simulink model "irp_model"  (R2016a)
settings: Solver=ode1  StartTime=0  StopTime=inf  FixedStep=0.001  RelTol=1e-3
PostLoadFcn:
  | , if any(exist('dsrtsu_mdlpostloadfcn', 'file') == [2, 3, 6]), try dsrtsu_mdlpostloadfcn('Execute', bdroot); catch fprintf('Error in PostLoadFcn (dsrtsu_mdlpostloadfcn) for model "%s":\n %s\n', bdroot, lasterr); end, end,
libraries: rtilibm x3, simulink_extras x3
settings Model: DSRTSU_INTERNAL_RTI_VER=460  DSRTSU_INTERNAL_RTI_TYPE=rti1005  DSRTSU_INTERNAL_RTIFPGA=50  Creator=k18w1400a  LastModifiedBy=Dominik
settings DataIOCC: LimitDataPoints=on  SaveFormat=Array
settings OptimizationCC: BlockReduction=off  BooleanDataType=off  OptimizeBlockIOStorage=off  BufferReuse=off  GlobalBufferReuse=off  ExpressionFolding=off  LocalBlockOutputs=off
settings HardwareCC: ProdBitPerPointer=32  ProdLargestAtomicFloat=None  ProdEndianess=BigEndian  ProdWordSize=32  ProdHWDeviceType=Generic->Custom  TargetIntDivRoundTo=Zero  TargetEndianess=BigEndian  TargetHWDeviceType=Generic->Custom
settings ModelReferenceCC: PropagateSignalLabelsOutOfModel=off
settings RTWCC: SystemTargetFile=rti1005.tlc  MakeCommand=make_rti  TemplateMakefile=rti1005.tmf  Description=dSPACE DS1005 Hardware Platform
settings STFCustomTargetCC: ParMdlRefBuildCompliant=on  GeneratePreprocessorConditionals=Disable all  SystemTargetFile=rti1005.tlc
settings GRTTargetCC: CompOptLevelCompliant=off  ConcurrentExecutionCompliant=off  CombineOutputUpdateFcns=off  MatFileLogging=off  CPPClassGenCompliant=off  GRTInterface=on  UseToolchainInfoCompliant=off  ExtModeMexFile=noextcomm
settings ConfigComp: CovModelRefEnable=Off

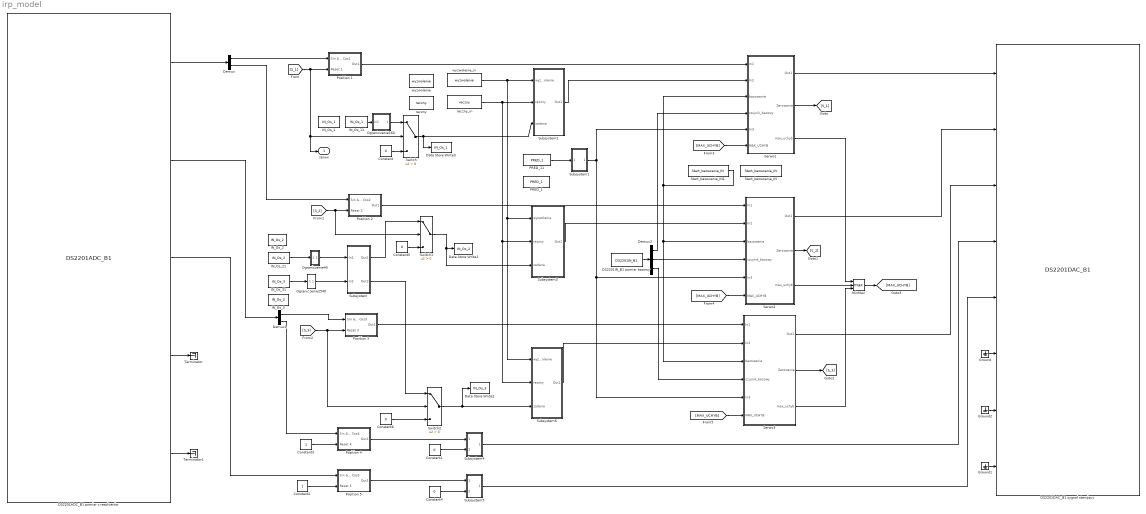
== system irp_model ==
  Constant{,1,4..6} (5 alike) : Constant  Value=0
  Constant2 : Constant
  Constant3 : Constant
  DS2201ADC_B1 pomiar z resolverów : rtilibm/DS2201/DS2201ADC_B1  BoardNo=1  channelNo1=[1 2 3 4]  channelNo2=[5 6 7 8]  channelNo3=[9 10]  channelNo4=-1  channelNo5=-1  DialogFcn=gui2201adc  UnitName={'DS2201ADC_B'}  UnitValues={ 1 }  DSProperties=struct('RTI',struct('Version',uint32(1),'BlockType',struct('isSLSource',uint8(1),'isSLSink',uint8(0),'isHWSource',uint8(1),'isHWSink',uint8(0),'isSetup',uint8(0),'isInline',uint8(1),'isNonInline',uint8(0),'isInterrupt',uint8(0),'isChannelwise',uint8(0)),'IOBoardType','DS2201','UnitType','ADC','Identifier','ADCMUX','DialogType','ML','BlockSet','NONE','SlaveProcessor','NONE'))
  DS2201DAC_B1 sygnał sterujący : rtilibm/DS2201/DS2201DAC_B1  BoardNo=1  IOErrorMode=[0 0]  InitValue=[0 0 0 0 0 0 0 0]  TermMode=[1 1 1 1 1 1 1 1]  TermValue=[0 0 0 0 0 0 0 0]  DialogFcn=gui2201dac  UnitName={'DS2201DAC_B'}  UnitValues={ 1 }  DSProperties=struct('RTI',struct('Version',uint32(1),'BlockType',struct('isSLSource',uint8(0),'isSLSink',uint8(1),'isHWSource',uint8(0),'isHWSink',uint8(1),'isSetup',uint8(0),'isInline',uint8(1),'isNonInline',uint8(0),'isInterrupt',uint8(0),'isChannelwise',uint8(0)),'IOBoardType','DS2201','UnitType','DAC','Identifier','DAC','DialogType','ML','BlockSet','NONE','SlaveProcessor','NONE'))
  DS2201IN_B1 pomiar bazowy : rtilibm/DS2201/DS2201IN_B1  BoardNo=1  ChannelNos=[1 2 3]  DialogFcn=gui2201in  UnitName={ 'DS2201IN_B' }  UnitValues={ 1 }  DSProperties=struct('RTI',struct('Version',uint32(1),'BlockType',struct('isSLSource',uint8(1),'isSLSink',uint8(0),'isHWSource',uint8(1),'isHWSink',uint8(0),'isSetup',uint8(0),'isInline',uint8(1),'isNonInline',uint8(0),'isInterrupt',uint8(0),'isChannelwise',uint8(0)),'IOBoardType','DS2201','UnitType','BIT','Identifier','BITIN','DialogType','ML','BlockSet','NONE','SlaveProcessor','NONE'))
  Data Store Write1 : DataStoreWrite  DataStoreName=IN_Os_2
  Data Store Write2 : DataStoreWrite  DataStoreName=IN_Os_3
  Data Store Write3 : DataStoreWrite  DataStoreName=IN_Os_1
  Demux : Demux  Outputs=2
  Demux1 : Demux  Outputs=2
  Demux2 : Demux  Outputs=3
  Ground : Ground
  Ground1 : Ground
  Ground2 : Ground
  "IN_Os_1 " : DataStoreMemory  DataStoreName=IN_Os_1  ReadBeforeWriteMsg=warning  WriteAfterWriteMsg=warning  WriteAfterReadMsg=warning  ShowAdditionalParam=off
  IN_Os_11 : DataStoreRead  DataStoreName=IN_Os_1
  "IN_Os_2 " : DataStoreMemory  DataStoreName=IN_Os_2  ReadBeforeWriteMsg=warning  WriteAfterWriteMsg=warning  WriteAfterReadMsg=warning  ShowAdditionalParam=off
  IN_Os_21 : DataStoreRead  DataStoreName=IN_Os_2
  "IN_Os_3 " : DataStoreMemory  DataStoreName=IN_Os_3  ReadBeforeWriteMsg=warning  WriteAfterWriteMsg=warning  WriteAfterReadMsg=warning  ShowAdditionalParam=off
  IN_Os_31 : DataStoreRead  DataStoreName=IN_Os_3
  MinMax : MinMax  Function=max  Inputs=3
  Ograniczenie160 : Subsystem
  Ograniczenie2540 : Subsystem
  Ograniczenie40 : Subsystem
  "PRED_1 " : DataStoreMemory  DataStoreName=PRED_1  ReadBeforeWriteMsg=warning  WriteAfterWriteMsg=warning  WriteAfterReadMsg=warning  InitialValue=50  ShowAdditionalParam=off
  "PRED_11 " : DataStoreRead  DataStoreName=PRED_1
  Position 1 : Subsystem
  Position 2 : Subsystem
  Position 3 : Subsystem
  Position 4 : Subsystem
  Position 5 : Subsystem
  Serwo1 : Subsystem
  Serwo2 : Subsystem
  Serwo3 : Subsystem
  "Start_bazowania_IN " : DataStoreMemory  DataStoreName=Start_bazowania_IN  ReadBeforeWriteMsg=warning  WriteAfterWriteMsg=warning  WriteAfterReadMsg=warning  ShowAdditionalParam=off
  Start_bazowania_IN1 : DataStoreRead  DataStoreName=Start_bazowania_IN
  Subsystem : Subsystem
  Subsystem1 : Subsystem
  Subsystem2 : Subsystem
  Subsystem3 : Subsystem
  Subsystem4 : Subsystem
  Subsystem5 : Subsystem
  Subsystem6 : Subsystem
  Switch : Switch  Criteria=u2 > Threshold
  Switch1 : Switch  Criteria=u2 > Threshold
  Switch2 : Switch  Criteria=u2 > Threshold
  Terminator : Terminator
  Terminator1 : Terminator
  "reczny " : DataStoreMemory  DataStoreName=reczny  ReadBeforeWriteMsg=warning  WriteAfterWriteMsg=warning  WriteAfterReadMsg=warning  ShowAdditionalParam=off
  "reczny_in " : DataStoreRead  DataStoreName=reczny
  "wyzwolenie " : DataStoreMemory  DataStoreName=wyzwolenie  ReadBeforeWriteMsg=warning  WriteAfterWriteMsg=warning  WriteAfterReadMsg=warning  ShowAdditionalParam=off
  "wyzwolenie_in " : DataStoreRead  DataStoreName=wyzwolenie
  zerow : Outport
  wires:
  Demux/1 -> Position 1/1(Sin && Cos1)
  Demux/2 -> Position 2/1(Sin && Cos2)
  DS2201ADC_B1 pomiar z resolverów/2 -> Demux1/1
  DS2201ADC_B1 pomiar z resolverów/1 -> Demux/1
  Demux1/1 -> Position 3/1(Sin && Cos3)
  Demux1/2 -> Position 4/1(Sin && Cos4)
  Constant3/1 -> Position 4/2(Reset 4)
  DS2201ADC_B1 pomiar z resolverów/3 -> Position 5/1(Sin && Cos5)
  Constant2/1 -> Position 5/2(Reset 5)
  IN_Os_21/1 -> Ograniczenie40/1(In1)
  IN_Os_31/1 -> Ograniczenie2540/1(In1)
  Ograniczenie40/1(Out1) -> Subsystem/1(In1)
  Ograniczenie2540/1(Out1) -> Subsystem/2(In2)
  Position 1/1(Out1) -> Serwo1/1(In1)
  Serwo1/1(Out1) -> DS2201DAC_B1 sygnał sterujący/1
  Serwo3/1(Out1) -> DS2201DAC_B1 sygnał sterujący/3
  Subsystem4/1(Out1) -> DS2201DAC_B1 sygnał sterujący/4
  Constant4/1 -> Subsystem5/2(In2)
  Subsystem5/1(Out1) -> DS2201DAC_B1 sygnał sterujący/5
  Start_bazowania_IN1/1 -> Serwo1/3(bazowanie), Serwo3/3(bazowanie), Serwo2/3(bazowanie)
  DS2201IN_B1 pomiar bazowy/1 -> Demux2/1
  Demux2/1 -> Serwo1/4(czujnik_bazowy)
  Serwo1/2(Zerowanie) -> [S_1]
  [S_1] -> zerow/1, Switch/2, Position 1/2(Reset 1)
  Position 2/1(Out1) -> Serwo2/1(In1)
  Demux2/2 -> Serwo2/4(czujnik_bazowy)
  Serwo2/2(Zerowanie) -> [S_2]
  Serwo2/1(Out1) -> DS2201DAC_B1 sygnał sterujący/2
  [S_2] -> Switch1/2, Position 2/2(Reset 2)
  Position 3/1(Out1) -> Serwo3/1(In1)
  Demux2/3 -> Serwo3/4(czujnik_bazowy)
  Serwo3/2(Zerowanie) -> [S_3]
  [S_3] -> Switch2/2, Position 3/2(Reset 3)
  Position 4/1(Out1) -> Subsystem4/1(In1)
  Position 5/1(Out1) -> Subsystem5/1(In1)
  Constant1/1 -> Subsystem4/2(In2)
  Ground/1 -> DS2201DAC_B1 sygnał sterujący/6
  Ground2/1 -> DS2201DAC_B1 sygnał sterujący/7
  Ground1/1 -> DS2201DAC_B1 sygnał sterujący/8
  DS2201ADC_B1 pomiar z resolverów/4 -> Terminator/1
  DS2201ADC_B1 pomiar z resolverów/5 -> Terminator1/1
  Ograniczenie160/1(Out1) -> Switch/1
  Constant/1 -> Switch/3
  Subsystem/1(Out1) -> Switch1/1
  Switch1/1 -> Subsystem3/3("zadana "), Data Store Write1/1
  Constant5/1 -> Switch1/3
  Subsystem/2(Out2) -> Switch2/1
  Constant6/1 -> Switch2/3
  "PRED_11 "/1 -> Subsystem1/1(In2)
  Subsystem1/1(Out1) -> Serwo1/5(In3), Serwo3/5(In3), Serwo2/5(In3)
  IN_Os_11/1 -> Ograniczenie160/1(In1)
  Switch/1 -> Data Store Write3/1, Subsystem2/3("zadana ")
  "wyzwolenie_in "/1 -> Subsystem6/1(wyzwolenie), Subsystem3/1(wyzwolenie), Subsystem2/1(wyzwolenie)
  "reczny_in "/1 -> Subsystem6/2("reczny "), Subsystem3/2("reczny "), Subsystem2/2("reczny ")
  Subsystem2/1(Out1) -> Serwo1/2(In2)
  Subsystem3/1(Out1) -> Serwo2/2(In2)
  Switch2/1 -> Data Store Write2/1, Subsystem6/3("zadana ")
  Subsystem6/1(Out1) -> Serwo3/2(In2)
  Serwo1/3("max_uchyb ") -> MinMax/1
  Serwo2/3("max_uchyb ") -> MinMax/2
  Serwo3/3("max_uchyb ") -> MinMax/3
  [MAX_UCHYB] -> Serwo1/6("MAX_UCHYB ")
  [MAX_UCHYB] -> Serwo2/6("MAX_UCHYB ")
  [MAX_UCHYB] -> Serwo3/6("MAX_UCHYB ")
  MinMax/1 -> [MAX_UCHYB]

== system irp_model/Ograniczenie160 ==
  In1 : Inport
  Abs : Abs
  Memory : Memory
  Switch : Switch  Criteria=u2 > Threshold  Threshold=160
  Out1 : Outport
  wires:
  In1/1 -> Switch/3, Abs/1
  Abs/1 -> Switch/2
  Switch/1 -> Memory/1, Out1/1
  Memory/1 -> Switch/1

== system irp_model/Ograniczenie2540 ==
  In1 : Inport
  Memory : Memory
  Memory1 : Memory
  Switch : Switch  Criteria=u2 > Threshold  Threshold=40
  Switch1 : Switch  Criteria=u2 > Threshold  Threshold=-25
  Out1 : Outport
  wires:
  In1/1 -> Switch1/1, Switch1/2
  Switch/1 -> Memory/1, Out1/1
  Switch1/1 -> Memory1/1, Switch/3, Switch/2
  Memory1/1 -> Switch1/3
  Memory/1 -> Switch/1

== system irp_model/Ograniczenie40 ==
  In1 : Inport
  Abs : Abs
  Memory : Memory
  Switch : Switch  Criteria=u2 > Threshold  Threshold=40
  Out1 : Outport
  wires:
  In1/1 -> Switch/3, Abs/1
  Abs/1 -> Switch/2
  Switch/1 -> Memory/1, Out1/1
  Memory/1 -> Switch/1

== system irp_model/Position 1 ==
  Sin && Cos1 : Inport
  Reset 1 : Inport  Port=2
  Filters 1 : Subsystem
  Position Calculation 1 : Subsystem
  Out1 : Outport
  wires:
  Filters 1/1(Sin) -> Position Calculation 1/1(Sin)
  Filters 1/2(Cos) -> Position Calculation 1/2(Cos)
  Sin && Cos1/1 -> Filters 1/1(Sin && Cos)
  Reset 1/1 -> Position Calculation 1/3(Reset (Impulse))
  Position Calculation 1/1(Position) -> Out1/1

== system irp_model/Position 2 ==
  Sin && Cos2 : Inport
  Reset 2 : Inport  Port=2
  Filters 2 : Subsystem
  Position Calculation 2 : Subsystem
  Out1 : Outport
  wires:
  Filters 2/1(Sin) -> Position Calculation 2/1(Sin)
  Filters 2/2(Cos) -> Position Calculation 2/2(Cos)
  Sin && Cos2/1 -> Filters 2/1(Sin && Cos)
  Reset 2/1 -> Position Calculation 2/3(Reset (Impulse))
  Position Calculation 2/1(Position) -> Out1/1

== system irp_model/Position 3 ==
  Sin && Cos3 : Inport
  Reset 3 : Inport  Port=2
  Filters 3 : Subsystem
  Position Calculation 3 : Subsystem
  Out1 : Outport
  wires:
  Filters 3/1(Sin) -> Position Calculation 3/1(Sin)
  Filters 3/2(Cos) -> Position Calculation 3/2(Cos)
  Sin && Cos3/1 -> Filters 3/1(Sin && Cos)
  Reset 3/1 -> Position Calculation 3/3(Reset (Impulse))
  Position Calculation 3/1(Position) -> Out1/1

== system irp_model/Position 4 ==
  Sin && Cos4 : Inport
  Reset 4 : Inport  Port=2
  Filters 4 : Subsystem
  Position Calculation 4 : Subsystem
  Out1 : Outport
  wires:
  Position Calculation 4/1(Position) -> Out1/1
  Reset 4/1 -> Position Calculation 4/3(Reset (Impulse))
  Sin && Cos4/1 -> Filters 4/1(Sin && Cos)
  Filters 4/2(Cos) -> Position Calculation 4/2(Cos)
  Filters 4/1(Sin) -> Position Calculation 4/1(Sin)

== system irp_model/Position 5 ==
  Sin && Cos5 : Inport
  Reset 5 : Inport  Port=2
  Filters 5 : Subsystem
  Position Calculation 5 : Subsystem
  Out1 : Outport
  wires:
  Position Calculation 5/1(Position) -> Out1/1
  Reset 5/1 -> Position Calculation 5/3(Reset (Impulse))
  Sin && Cos5/1 -> Filters 5/1(Sin && Cos)
  Filters 5/2(Cos) -> Position Calculation 5/2(Cos)
  Filters 5/1(Sin) -> Position Calculation 5/1(Sin)

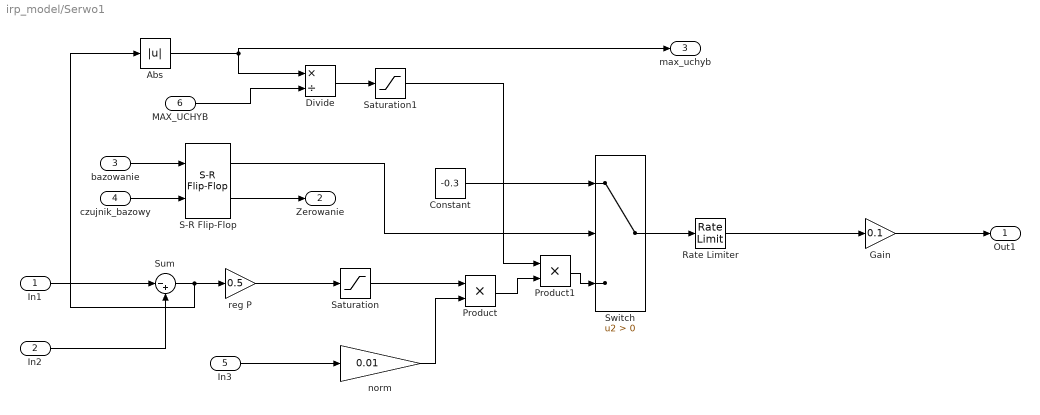
== system irp_model/Serwo1 ==
  In1 : Inport
  In2 : Inport  Port=2
  bazowanie : Inport  Port=3
  czujnik_bazowy : Inport  Port=4
  In3 : Inport  Port=5
  "MAX_UCHYB " : Inport  Port=6
  Abs : Abs
  Constant : Constant  Value=-0.3
  Divide : Product  Inputs=*/
  Gain : Gain  Gain=0.1
  Product : Product
  Product1 : Product
  Rate Limiter : RateLimiter  RisingSlewLimit=50  FallingSlewLimit=-50  SampleTimeMode=inherited
  S-R Flip-Flop : simulink_extras/Flip Flops/S-R Flip-Flop  initial_condition=0
  Saturation : Saturate  UpperLimit=3  LowerLimit=-3
  Saturation1 : Saturate  UpperLimit=1  LowerLimit=0.001
  Sum : Sum  Inputs=|-+
  Switch : Switch  Criteria=u2 > Threshold
  norm : Gain  Gain=0.01
  reg P : Gain  Gain=0.5
  Out1 : Outport
  Zerowanie : Outport  Port=2
  "max_uchyb " : Outport  Port=3
  wires:
  Rate Limiter/1 -> Gain/1
  Gain/1 -> Out1/1
  In1/1 -> Sum/1
  Sum/1 -> Abs/1, reg P/1
  reg P/1 -> Saturation/1
  In2/1 -> Sum/2
  Constant/1 -> Switch/1
  Switch/1 -> Rate Limiter/1
  S-R Flip-Flop/2 -> Zerowanie/1
  czujnik_bazowy/1 -> S-R Flip-Flop/2
  bazowanie/1 -> S-R Flip-Flop/1
  S-R Flip-Flop/1 -> Switch/2
  Saturation/1 -> Product/1
  norm/1 -> Product/2
  In3/1 -> norm/1
  Abs/1 -> Divide/1, "max_uchyb "/1
  Divide/1 -> Saturation1/1
  Product/1 -> Product1/2
  Saturation1/1 -> Product1/1
  "MAX_UCHYB "/1 -> Divide/2
  Product1/1 -> Switch/3

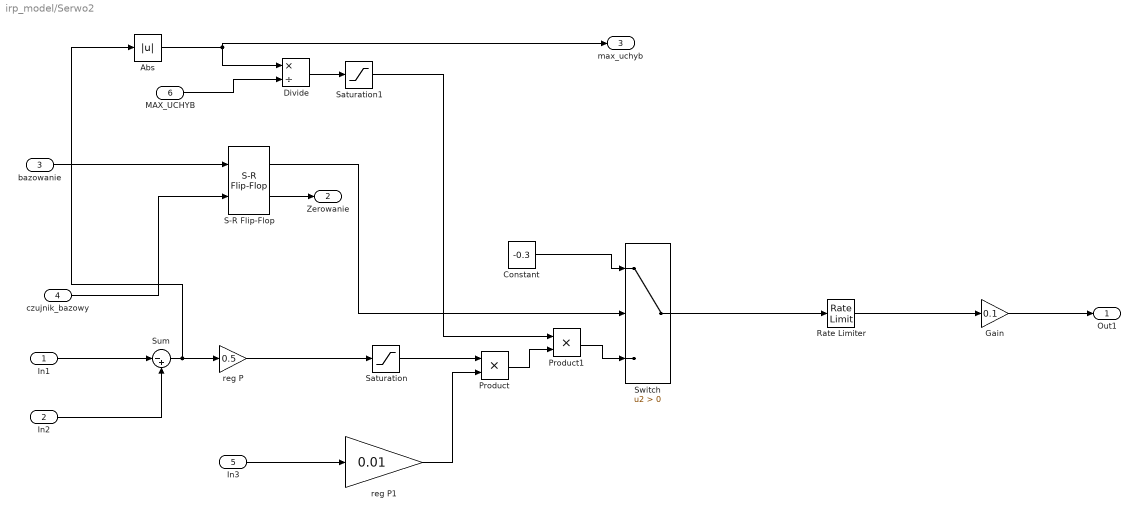
== system irp_model/Serwo2 ==
  In1 : Inport
  In2 : Inport  Port=2
  bazowanie : Inport  Port=3
  czujnik_bazowy : Inport  Port=4
  In3 : Inport  Port=5
  "MAX_UCHYB " : Inport  Port=6
  Abs : Abs
  Constant : Constant  Value=-0.3
  Divide : Product  Inputs=*/
  Gain : Gain  Gain=0.1
  Product : Product
  Product1 : Product
  Rate Limiter : RateLimiter  RisingSlewLimit=50  FallingSlewLimit=-50  SampleTimeMode=inherited
  S-R Flip-Flop : simulink_extras/Flip Flops/S-R Flip-Flop  initial_condition=0
  Saturation : Saturate  UpperLimit=3  LowerLimit=-3
  Saturation1 : Saturate  UpperLimit=1  LowerLimit=0.001
  Sum : Sum  Inputs=|-+
  Switch : Switch  Criteria=u2 > Threshold
  reg P : Gain  Gain=0.5
  reg P1 : Gain  Gain=0.01
  Out1 : Outport
  Zerowanie : Outport  Port=2
  "max_uchyb " : Outport  Port=3
  wires:
  Rate Limiter/1 -> Gain/1
  Gain/1 -> Out1/1
  In1/1 -> Sum/1
  reg P/1 -> Saturation/1
  In2/1 -> Sum/2
  Constant/1 -> Switch/1
  Switch/1 -> Rate Limiter/1
  S-R Flip-Flop/2 -> Zerowanie/1
  czujnik_bazowy/1 -> S-R Flip-Flop/2
  bazowanie/1 -> S-R Flip-Flop/1
  S-R Flip-Flop/1 -> Switch/2
  Saturation/1 -> Product/1
  In3/1 -> reg P1/1
  reg P1/1 -> Product/2
  Sum/1 -> reg P/1, Abs/1
  Abs/1 -> "max_uchyb "/1, Divide/1
  Divide/1 -> Saturation1/1
  Saturation1/1 -> Product1/1
  "MAX_UCHYB "/1 -> Divide/2
  Product/1 -> Product1/2
  Product1/1 -> Switch/3

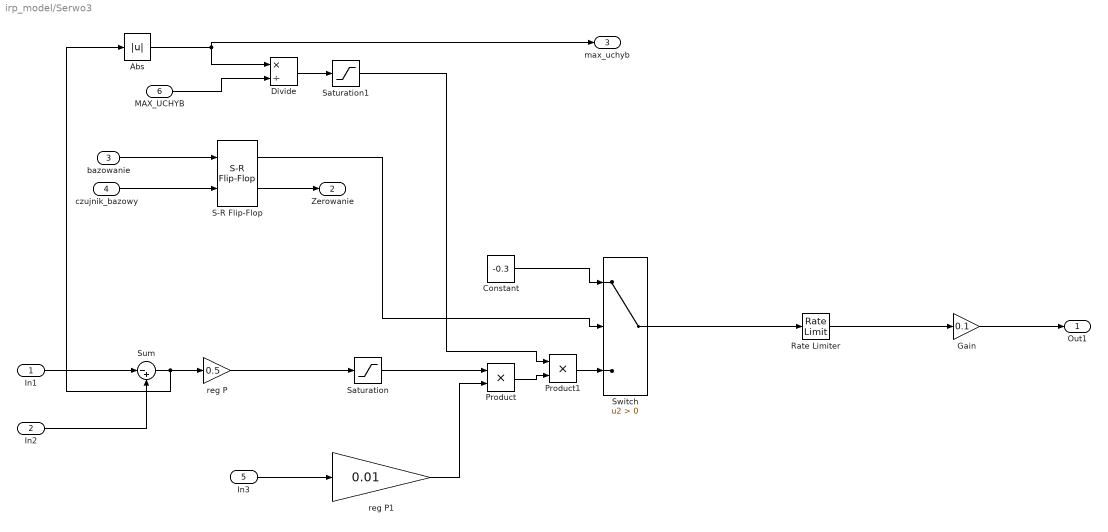
== system irp_model/Serwo3 ==
  In1 : Inport
  In2 : Inport  Port=2
  bazowanie : Inport  Port=3
  czujnik_bazowy : Inport  Port=4
  In3 : Inport  Port=5
  "MAX_UCHYB " : Inport  Port=6
  Abs : Abs
  Constant : Constant  Value=-0.3
  Divide : Product  Inputs=*/
  Gain : Gain  Gain=0.1
  Product : Product
  Product1 : Product
  Rate Limiter : RateLimiter  RisingSlewLimit=50  FallingSlewLimit=-50  SampleTimeMode=inherited
  S-R Flip-Flop : simulink_extras/Flip Flops/S-R Flip-Flop  initial_condition=0
  Saturation : Saturate  UpperLimit=3  LowerLimit=-3
  Saturation1 : Saturate  UpperLimit=1  LowerLimit=0.001
  Sum : Sum  Inputs=|-+
  Switch : Switch  Criteria=u2 > Threshold
  reg P : Gain  Gain=0.5
  reg P1 : Gain  Gain=0.01
  Out1 : Outport
  Zerowanie : Outport  Port=2
  "max_uchyb " : Outport  Port=3
  wires:
  Rate Limiter/1 -> Gain/1
  Gain/1 -> Out1/1
  In1/1 -> Sum/1
  reg P/1 -> Saturation/1
  In2/1 -> Sum/2
  czujnik_bazowy/1 -> S-R Flip-Flop/2
  Constant/1 -> Switch/1
  Switch/1 -> Rate Limiter/1
  bazowanie/1 -> S-R Flip-Flop/1
  S-R Flip-Flop/2 -> Zerowanie/1
  S-R Flip-Flop/1 -> Switch/2
  Saturation/1 -> Product/1
  reg P1/1 -> Product/2
  In3/1 -> reg P1/1
  Abs/1 -> Divide/1, "max_uchyb "/1
  Divide/1 -> Saturation1/1
  Saturation1/1 -> Product1/1
  "MAX_UCHYB "/1 -> Divide/2
  Sum/1 -> Abs/1, reg P/1
  Product/1 -> Product1/2
  Product1/1 -> Switch/3

== system irp_model/Subsystem ==
  In1 : Inport
  In2 : Inport  Port=2
  Abs : Abs
  Constant : Constant
  Constant1 : Constant  Value=0
  Memory : Memory
  Memory1 : Memory
  Sum3 : Sum  Inputs=|-+
  Switch : Switch  Criteria=u2 > Threshold  Threshold=40
  Switch1 : Switch  Criteria=u2 > Threshold
  Switch2 : Switch  Criteria=u2 > Threshold
  Out1 : Outport
  Out2 : Outport  Port=2
  wires:
  In2/1 -> Switch1/1, Sum3/2
  In1/1 -> Switch2/1, Sum3/1
  Sum3/1 -> Abs/1
  Abs/1 -> Switch/2
  Switch2/1 -> Memory1/1, Out1/1
  Switch/1 -> Switch1/2, Switch2/2
  Memory1/1 -> Switch2/3
  Switch1/1 -> Out2/1, Memory/1
  Memory/1 -> Switch1/3
  Constant/1 -> Switch/3
  Constant1/1 -> Switch/1

== system irp_model/Subsystem1 ==
  In2 : Inport
  Memory : Memory
  Memory1 : Memory
  Switch3 : Switch  Threshold=100
  Switch4 : Switch  Criteria=u2 > Threshold  Threshold=1
  Out1 : Outport
  wires:
  Switch4/1 -> Memory1/1, Switch3/3, Switch3/2
  Memory1/1 -> Switch4/3
  Switch3/1 -> Memory/1, Out1/1
  In2/1 -> Switch4/1, Switch4/2
  Memory/1 -> Switch3/1

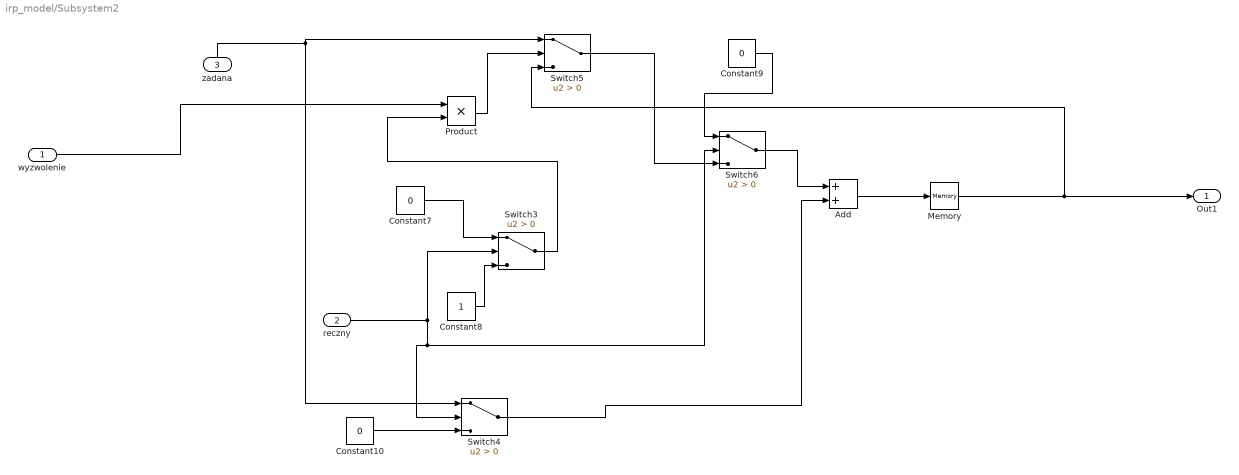
== system irp_model/Subsystem2 ==
  wyzwolenie : Inport
  "reczny " : Inport  Port=2
  "zadana " : Inport  Port=3
  Add : Sum
  Constant10 : Constant  Value=0
  Constant7 : Constant  Value=0
  Constant8 : Constant
  Constant9 : Constant  Value=0
  Memory : Memory
  Product : Product
  Switch{3..6} (4 alike) : Switch  Criteria=u2 > Threshold
  Out1 : Outport
  wires:
  Constant7/1 -> Switch3/1
  Switch4/1 -> Add/2
  "reczny "/1 -> Switch3/2, Switch4/2, Switch6/2
  wyzwolenie/1 -> Product/1
  Add/1 -> Memory/1
  Product/1 -> Switch5/2
  Switch5/1 -> Switch6/3
  "zadana "/1 -> Switch4/1, Switch5/1
  Memory/1 -> Out1/1, Switch5/3
  Constant8/1 -> Switch3/3
  Constant9/1 -> Switch6/1
  Constant10/1 -> Switch4/3
  Switch3/1 -> Product/2
  Switch6/1 -> Add/1

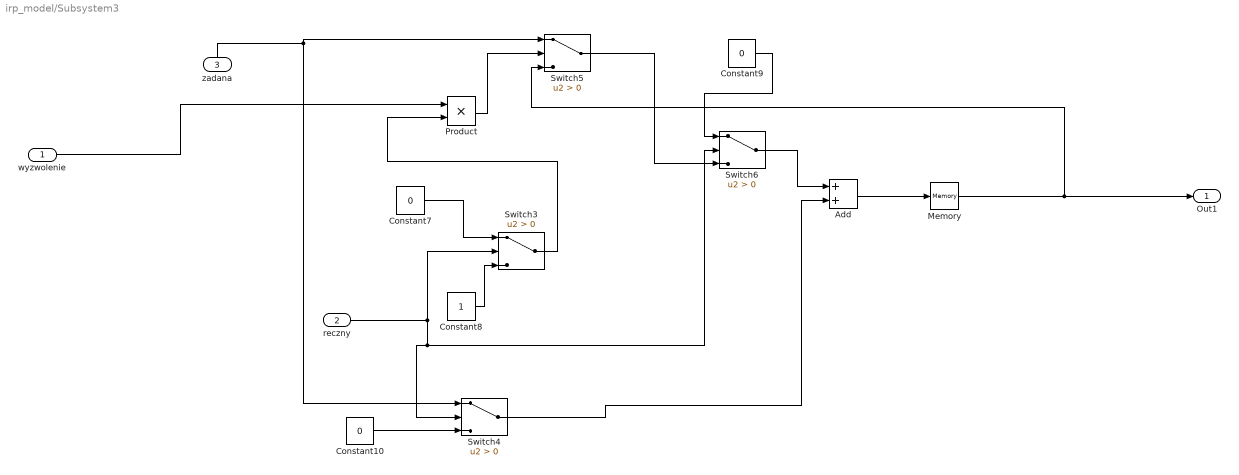
== system irp_model/Subsystem3 ==
  wyzwolenie : Inport
  "reczny " : Inport  Port=2
  "zadana " : Inport  Port=3
  Add : Sum
  Constant10 : Constant  Value=0
  Constant7 : Constant  Value=0
  Constant8 : Constant
  Constant9 : Constant  Value=0
  Memory : Memory
  Product : Product
  Switch{3..6} (4 alike) : Switch  Criteria=u2 > Threshold
  Out1 : Outport
  wires:
  Constant7/1 -> Switch3/1
  Switch4/1 -> Add/2
  "reczny "/1 -> Switch3/2, Switch4/2, Switch6/2
  wyzwolenie/1 -> Product/1
  Add/1 -> Memory/1
  Product/1 -> Switch5/2
  Switch5/1 -> Switch6/3
  "zadana "/1 -> Switch4/1, Switch5/1
  Memory/1 -> Out1/1, Switch5/3
  Constant8/1 -> Switch3/3
  Constant9/1 -> Switch6/1
  Constant10/1 -> Switch4/3
  Switch3/1 -> Product/2
  Switch6/1 -> Add/1

== system irp_model/Subsystem4 ==
  In1 : Inport
  In2 : Inport  Port=2
  Gain4 : Gain  Gain=0.1
  Rate Limiter4 : RateLimiter  RisingSlewLimit=50  FallingSlewLimit=-50  SampleTimeMode=inherited
  Saturation4 : Saturate  UpperLimit=3  LowerLimit=-3
  Sum3 : Sum  Inputs=|-+
  reg P4 : Gain  Gain=0.5
  Out1 : Outport
  wires:
  Saturation4/1 -> Rate Limiter4/1
  In2/1 -> Sum3/2
  Rate Limiter4/1 -> Gain4/1
  reg P4/1 -> Saturation4/1
  Sum3/1 -> reg P4/1
  Gain4/1 -> Out1/1
  In1/1 -> Sum3/1

== system irp_model/Subsystem5 ==
  In1 : Inport
  In2 : Inport  Port=2
  Gain3 : Gain  Gain=0.1
  Rate Limiter3 : RateLimiter  RisingSlewLimit=50  FallingSlewLimit=-50  SampleTimeMode=inherited
  Saturation3 : Saturate  UpperLimit=3  LowerLimit=-3
  Sum4 : Sum  Inputs=|-+
  reg P3 : Gain  Gain=0.5
  Out1 : Outport
  wires:
  Gain3/1 -> Out1/1
  Saturation3/1 -> Rate Limiter3/1
  Sum4/1 -> reg P3/1
  Rate Limiter3/1 -> Gain3/1
  In2/1 -> Sum4/2
  reg P3/1 -> Saturation3/1
  In1/1 -> Sum4/1

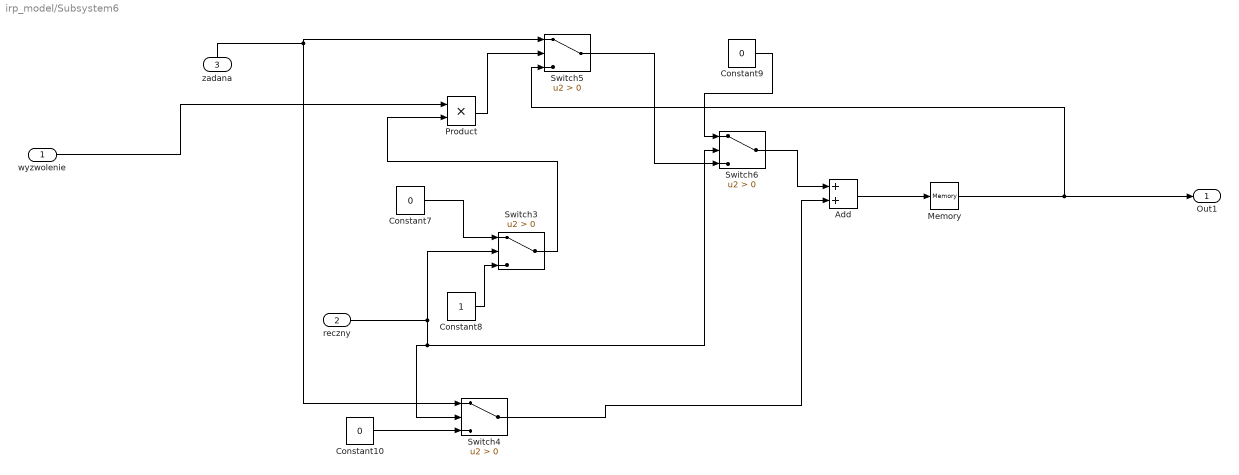
== system irp_model/Subsystem6 ==
  wyzwolenie : Inport
  "reczny " : Inport  Port=2
  "zadana " : Inport  Port=3
  Add : Sum
  Constant10 : Constant  Value=0
  Constant7 : Constant  Value=0
  Constant8 : Constant
  Constant9 : Constant  Value=0
  Memory : Memory
  Product : Product
  Switch{3..6} (4 alike) : Switch  Criteria=u2 > Threshold
  Out1 : Outport
  wires:
  Constant7/1 -> Switch3/1
  Switch4/1 -> Add/2
  "reczny "/1 -> Switch3/2, Switch4/2, Switch6/2
  wyzwolenie/1 -> Product/1
  Add/1 -> Memory/1
  Product/1 -> Switch5/2
  Switch5/1 -> Switch6/3
  "zadana "/1 -> Switch4/1, Switch5/1
  Memory/1 -> Out1/1, Switch5/3
  Constant8/1 -> Switch3/3
  Constant9/1 -> Switch6/1
  Constant10/1 -> Switch4/3
  Switch3/1 -> Product/2
  Switch6/1 -> Add/1

== system irp_model/Position 1/Filters 1 ==
  Sin && Cos : Inport
  Analog Butterworth LP Filter : Subsystem  mask(buttap){}
      mask help:
      | Analog Butterworth low pass filter.
      |
      | (Requires Signal Processing Toolbox)
      mask init:
      | [z,p,k]=buttap(@2); z=@1*z; p=@1*p; k=real(prod(-p)); [num,den]=zp2tf(z,p,k); w=logspace(log10(@1/10),log10(10*@1),20); h=freqs(num,den,w);
      mask Help: Butterworth low pass filter using MATLAB's butter command.
      mask Display: plot(20*log10(w),20*log10(abs(h)))
  Analog Butterworth LP Filter1 : Subsystem  mask(buttap){}
      mask help:
      | Analog Butterworth low pass filter.
      |
      | (Requires Signal Processing Toolbox)
      mask init:
      | [z,p,k]=buttap(@2); z=@1*z; p=@1*p; k=real(prod(-p)); [num,den]=zp2tf(z,p,k); w=logspace(log10(@1/10),log10(10*@1),20); h=freqs(num,den,w);
      mask Help: Butterworth low pass filter using MATLAB's butter command.
      mask Display: plot(20*log10(w),20*log10(abs(h)))
  Demux : Demux  Outputs=2
  Sin : Outport
  Cos : Outport  Port=2
  wires:
  Demux/2 -> Analog Butterworth LP Filter1/1(In1)
  Demux/1 -> Analog Butterworth LP Filter/1(In1)
  Sin && Cos/1 -> Demux/1
  Analog Butterworth LP Filter1/1(Out1) -> Cos/1
  Analog Butterworth LP Filter/1(Out1) -> Sin/1

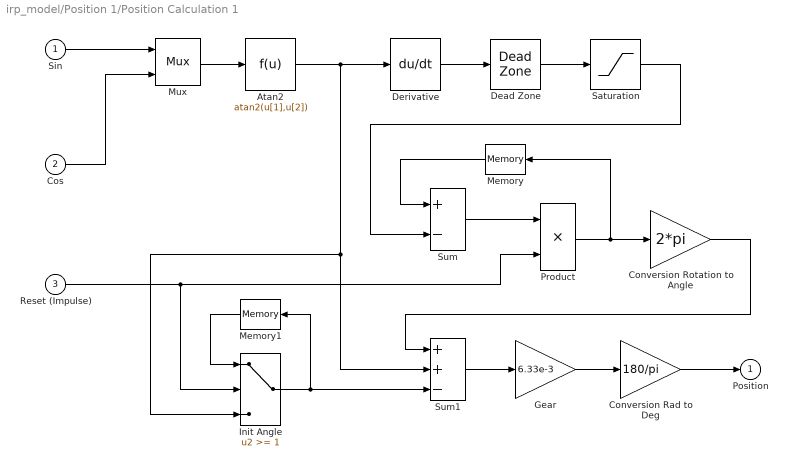
== system irp_model/Position 1/Position Calculation 1 ==
  Sin : Inport
  Cos : Inport  Port=2
  Reset (Impulse) : Inport  Port=3
  Atan2 : Fcn  Expr=atan2(u[1],u[2])
  Conversion Rad to Deg : Gain  Gain=180/pi  SaturateOnIntegerOverflow=on  OutDataTypeStr=Inherit: Same as input  ParamDataTypeStr=Inherit: Same as input
  Conversion Rotation to Angle : Gain  Gain=2*pi  SaturateOnIntegerOverflow=on  OutDataTypeStr=Inherit: Same as input  ParamDataTypeStr=Inherit: Same as input
  Dead Zone : DeadZone  LowerValue=-5000  UpperValue=5000  SaturateOnIntegerOverflow=on
  Derivative : Derivative
  Gear : Gain  Gain=6.33e-3  SaturateOnIntegerOverflow=on  OutDataTypeStr=Inherit: Same as input  ParamDataTypeStr=Inherit: Same as input
  Init Angle : Switch  Threshold=1  SaturateOnIntegerOverflow=on  InputSameDT=on
  Memory : Memory
  Memory1 : Memory
  Mux : Mux  Inputs=2
  Product : Product  SaturateOnIntegerOverflow=on  RndMeth=Zero  InputSameDT=on  OutDataTypeStr=Inherit: Same as first input
  Saturation : Saturate  UpperLimit=1  LowerLimit=-1
  Sum : Sum  Inputs=+-  SaturateOnIntegerOverflow=on  InputSameDT=on  OutDataTypeStr=Inherit: Same as first input
  Sum1 : Sum  Inputs=++-  SaturateOnIntegerOverflow=on  InputSameDT=on  OutDataTypeStr=Inherit: Same as first input
  Position : Outport
  wires:
  Init Angle/1 -> Memory1/1, Sum1/3
  Memory1/1 -> Init Angle/1
  Product/1 -> Memory/1, Conversion Rotation to Angle/1
  Memory/1 -> Sum/1
  Cos/1 -> Mux/2
  Atan2/1 -> Init Angle/3, Sum1/2, Derivative/1
  Reset (Impulse)/1 -> Init Angle/2, Product/2
  Conversion Rotation to Angle/1 -> Sum1/1
  Saturation/1 -> Sum/2
  Conversion Rad to Deg/1 -> Position/1
  Sin/1 -> Mux/1
  Mux/1 -> Atan2/1
  Derivative/1 -> Dead Zone/1
  Dead Zone/1 -> Saturation/1
  Sum/1 -> Product/1
  Sum1/1 -> Gear/1
  Gear/1 -> Conversion Rad to Deg/1

== system irp_model/Position 2/Filters 2 ==
  Sin && Cos : Inport
  Analog Butterworth LP Filter : Subsystem  mask(buttap){}
      mask help:
      | Analog Butterworth low pass filter.
      |
      | (Requires Signal Processing Toolbox)
      mask init:
      | [z,p,k]=buttap(@2); z=@1*z; p=@1*p; k=real(prod(-p)); [num,den]=zp2tf(z,p,k); w=logspace(log10(@1/10),log10(10*@1),20); h=freqs(num,den,w);
      mask Help: Butterworth low pass filter using MATLAB's butter command.
      mask Display: plot(20*log10(w),20*log10(abs(h)))
  Analog Butterworth LP Filter1 : Subsystem  mask(buttap){}
      mask help:
      | Analog Butterworth low pass filter.
      |
      | (Requires Signal Processing Toolbox)
      mask init:
      | [z,p,k]=buttap(@2); z=@1*z; p=@1*p; k=real(prod(-p)); [num,den]=zp2tf(z,p,k); w=logspace(log10(@1/10),log10(10*@1),20); h=freqs(num,den,w);
      mask Help: Butterworth low pass filter using MATLAB's butter command.
      mask Display: plot(20*log10(w),20*log10(abs(h)))
  Demux : Demux  Outputs=2
  Sin : Outport
  Cos : Outport  Port=2
  wires:
  Demux/2 -> Analog Butterworth LP Filter1/1(In1)
  Demux/1 -> Analog Butterworth LP Filter/1(In1)
  Sin && Cos/1 -> Demux/1
  Analog Butterworth LP Filter1/1(Out1) -> Cos/1
  Analog Butterworth LP Filter/1(Out1) -> Sin/1

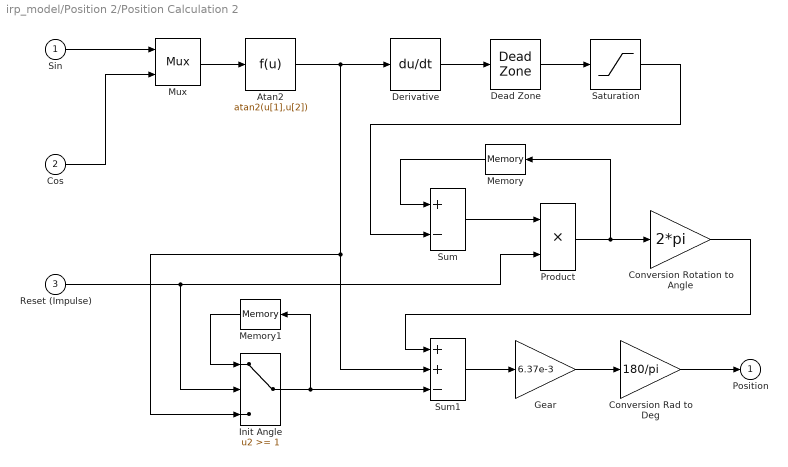
== system irp_model/Position 2/Position Calculation 2 ==
  Sin : Inport
  Cos : Inport  Port=2
  Reset (Impulse) : Inport  Port=3
  Atan2 : Fcn  Expr=atan2(u[1],u[2])
  Conversion Rad to Deg : Gain  Gain=180/pi  SaturateOnIntegerOverflow=on  OutDataTypeStr=Inherit: Same as input  ParamDataTypeStr=Inherit: Same as input
  Conversion Rotation to Angle : Gain  Gain=2*pi  SaturateOnIntegerOverflow=on  OutDataTypeStr=Inherit: Same as input  ParamDataTypeStr=Inherit: Same as input
  Dead Zone : DeadZone  LowerValue=-5000  UpperValue=5000  SaturateOnIntegerOverflow=on
  Derivative : Derivative
  Gear : Gain  Gain=6.37e-3  SaturateOnIntegerOverflow=on  OutDataTypeStr=Inherit: Same as input  ParamDataTypeStr=Inherit: Same as input
  Init Angle : Switch  Threshold=1  SaturateOnIntegerOverflow=on  InputSameDT=on
  Memory : Memory
  Memory1 : Memory
  Mux : Mux  Inputs=2
  Product : Product  SaturateOnIntegerOverflow=on  RndMeth=Zero  InputSameDT=on  OutDataTypeStr=Inherit: Same as first input
  Saturation : Saturate  UpperLimit=1  LowerLimit=-1
  Sum : Sum  Inputs=+-  SaturateOnIntegerOverflow=on  InputSameDT=on  OutDataTypeStr=Inherit: Same as first input
  Sum1 : Sum  Inputs=++-  SaturateOnIntegerOverflow=on  InputSameDT=on  OutDataTypeStr=Inherit: Same as first input
  Position : Outport
  wires:
  Init Angle/1 -> Memory1/1, Sum1/3
  Memory1/1 -> Init Angle/1
  Product/1 -> Memory/1, Conversion Rotation to Angle/1
  Memory/1 -> Sum/1
  Cos/1 -> Mux/2
  Atan2/1 -> Init Angle/3, Sum1/2, Derivative/1
  Reset (Impulse)/1 -> Init Angle/2, Product/2
  Conversion Rotation to Angle/1 -> Sum1/1
  Saturation/1 -> Sum/2
  Conversion Rad to Deg/1 -> Position/1
  Sin/1 -> Mux/1
  Mux/1 -> Atan2/1
  Derivative/1 -> Dead Zone/1
  Dead Zone/1 -> Saturation/1
  Sum/1 -> Product/1
  Sum1/1 -> Gear/1
  Gear/1 -> Conversion Rad to Deg/1

== system irp_model/Position 3/Filters 3 ==
  Sin && Cos : Inport
  Analog Butterworth LP Filter : Subsystem  mask(buttap){}
      mask help:
      | Analog Butterworth low pass filter.
      |
      | (Requires Signal Processing Toolbox)
      mask init:
      | [z,p,k]=buttap(@2); z=@1*z; p=@1*p; k=real(prod(-p)); [num,den]=zp2tf(z,p,k); w=logspace(log10(@1/10),log10(10*@1),20); h=freqs(num,den,w);
      mask Help: Butterworth low pass filter using MATLAB's butter command.
      mask Display: plot(20*log10(w),20*log10(abs(h)))
  Analog Butterworth LP Filter1 : Subsystem  mask(buttap){}
      mask help:
      | Analog Butterworth low pass filter.
      |
      | (Requires Signal Processing Toolbox)
      mask init:
      | [z,p,k]=buttap(@2); z=@1*z; p=@1*p; k=real(prod(-p)); [num,den]=zp2tf(z,p,k); w=logspace(log10(@1/10),log10(10*@1),20); h=freqs(num,den,w);
      mask Help: Butterworth low pass filter using MATLAB's butter command.
      mask Display: plot(20*log10(w),20*log10(abs(h)))
  Demux : Demux  Outputs=2
  Sin : Outport
  Cos : Outport  Port=2
  wires:
  Demux/2 -> Analog Butterworth LP Filter1/1(In1)
  Demux/1 -> Analog Butterworth LP Filter/1(In1)
  Sin && Cos/1 -> Demux/1
  Analog Butterworth LP Filter1/1(Out1) -> Cos/1
  Analog Butterworth LP Filter/1(Out1) -> Sin/1

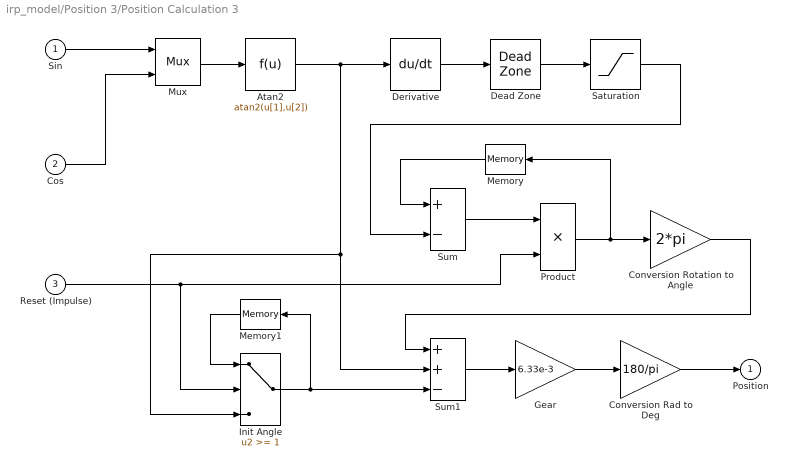
== system irp_model/Position 3/Position Calculation 3 ==
  Sin : Inport
  Cos : Inport  Port=2
  Reset (Impulse) : Inport  Port=3
  Atan2 : Fcn  Expr=atan2(u[1],u[2])
  Conversion Rad to Deg : Gain  Gain=180/pi  SaturateOnIntegerOverflow=on  OutDataTypeStr=Inherit: Same as input  ParamDataTypeStr=Inherit: Same as input
  Conversion Rotation to Angle : Gain  Gain=2*pi  SaturateOnIntegerOverflow=on  OutDataTypeStr=Inherit: Same as input  ParamDataTypeStr=Inherit: Same as input
  Dead Zone : DeadZone  LowerValue=-5000  UpperValue=5000  SaturateOnIntegerOverflow=on
  Derivative : Derivative
  Gear : Gain  Gain=6.33e-3  SaturateOnIntegerOverflow=on  OutDataTypeStr=Inherit: Same as input  ParamDataTypeStr=Inherit: Same as input
  Init Angle : Switch  Threshold=1  SaturateOnIntegerOverflow=on  InputSameDT=on
  Memory : Memory
  Memory1 : Memory
  Mux : Mux  Inputs=2
  Product : Product  SaturateOnIntegerOverflow=on  RndMeth=Zero  InputSameDT=on  OutDataTypeStr=Inherit: Same as first input
  Saturation : Saturate  UpperLimit=1  LowerLimit=-1
  Sum : Sum  Inputs=+-  SaturateOnIntegerOverflow=on  InputSameDT=on  OutDataTypeStr=Inherit: Same as first input
  Sum1 : Sum  Inputs=++-  SaturateOnIntegerOverflow=on  InputSameDT=on  OutDataTypeStr=Inherit: Same as first input
  Position : Outport
  wires:
  Init Angle/1 -> Memory1/1, Sum1/3
  Memory1/1 -> Init Angle/1
  Product/1 -> Memory/1, Conversion Rotation to Angle/1
  Memory/1 -> Sum/1
  Cos/1 -> Mux/2
  Atan2/1 -> Init Angle/3, Sum1/2, Derivative/1
  Reset (Impulse)/1 -> Init Angle/2, Product/2
  Conversion Rotation to Angle/1 -> Sum1/1
  Saturation/1 -> Sum/2
  Conversion Rad to Deg/1 -> Position/1
  Sin/1 -> Mux/1
  Mux/1 -> Atan2/1
  Derivative/1 -> Dead Zone/1
  Dead Zone/1 -> Saturation/1
  Sum/1 -> Product/1
  Sum1/1 -> Gear/1
  Gear/1 -> Conversion Rad to Deg/1

== system irp_model/Position 4/Filters 4 ==
  Sin && Cos : Inport
  Analog Butterworth LP Filter : Subsystem  mask(buttap){}
      mask help:
      | Analog Butterworth low pass filter.
      |
      | (Requires Signal Processing Toolbox)
      mask init:
      | [z,p,k]=buttap(@2); z=@1*z; p=@1*p; k=real(prod(-p)); [num,den]=zp2tf(z,p,k); w=logspace(log10(@1/10),log10(10*@1),20); h=freqs(num,den,w);
      mask Help: Butterworth low pass filter using MATLAB's butter command.
      mask Display: plot(20*log10(w),20*log10(abs(h)))
  Analog Butterworth LP Filter1 : Subsystem  mask(buttap){}
      mask help:
      | Analog Butterworth low pass filter.
      |
      | (Requires Signal Processing Toolbox)
      mask init:
      | [z,p,k]=buttap(@2); z=@1*z; p=@1*p; k=real(prod(-p)); [num,den]=zp2tf(z,p,k); w=logspace(log10(@1/10),log10(10*@1),20); h=freqs(num,den,w);
      mask Help: Butterworth low pass filter using MATLAB's butter command.
      mask Display: plot(20*log10(w),20*log10(abs(h)))
  Demux : Demux  Outputs=2
  Sin : Outport
  Cos : Outport  Port=2
  wires:
  Analog Butterworth LP Filter/1(Out1) -> Sin/1
  Analog Butterworth LP Filter1/1(Out1) -> Cos/1
  Sin && Cos/1 -> Demux/1
  Demux/1 -> Analog Butterworth LP Filter/1(In1)
  Demux/2 -> Analog Butterworth LP Filter1/1(In1)

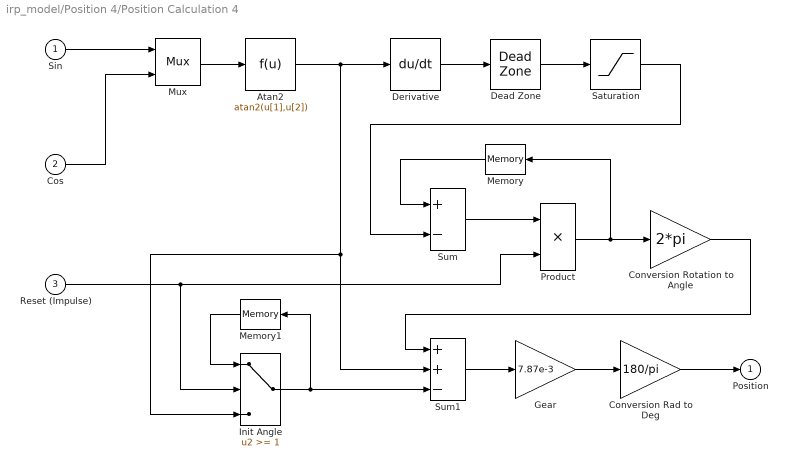
== system irp_model/Position 4/Position Calculation 4 ==
  Sin : Inport
  Cos : Inport  Port=2
  Reset (Impulse) : Inport  Port=3
  Atan2 : Fcn  Expr=atan2(u[1],u[2])
  Conversion Rad to Deg : Gain  Gain=180/pi  SaturateOnIntegerOverflow=on  OutDataTypeStr=Inherit: Same as input  ParamDataTypeStr=Inherit: Same as input
  Conversion Rotation to Angle : Gain  Gain=2*pi  SaturateOnIntegerOverflow=on  OutDataTypeStr=Inherit: Same as input  ParamDataTypeStr=Inherit: Same as input
  Dead Zone : DeadZone  LowerValue=-5000  UpperValue=5000  SaturateOnIntegerOverflow=on
  Derivative : Derivative
  Gear : Gain  Gain=7.87e-3  SaturateOnIntegerOverflow=on  OutDataTypeStr=Inherit: Same as input  ParamDataTypeStr=Inherit: Same as input
  Init Angle : Switch  Threshold=1  SaturateOnIntegerOverflow=on  InputSameDT=on
  Memory : Memory
  Memory1 : Memory
  Mux : Mux  Inputs=2
  Product : Product  SaturateOnIntegerOverflow=on  RndMeth=Zero  InputSameDT=on  OutDataTypeStr=Inherit: Same as first input
  Saturation : Saturate  UpperLimit=1  LowerLimit=-1
  Sum : Sum  Inputs=+-  SaturateOnIntegerOverflow=on  InputSameDT=on  OutDataTypeStr=Inherit: Same as first input
  Sum1 : Sum  Inputs=++-  SaturateOnIntegerOverflow=on  InputSameDT=on  OutDataTypeStr=Inherit: Same as first input
  Position : Outport
  wires:
  Gear/1 -> Conversion Rad to Deg/1
  Sum1/1 -> Gear/1
  Sum/1 -> Product/1
  Dead Zone/1 -> Saturation/1
  Derivative/1 -> Dead Zone/1
  Mux/1 -> Atan2/1
  Sin/1 -> Mux/1
  Conversion Rad to Deg/1 -> Position/1
  Saturation/1 -> Sum/2
  Conversion Rotation to Angle/1 -> Sum1/1
  Reset (Impulse)/1 -> Product/2, Init Angle/2
  Atan2/1 -> Derivative/1, Sum1/2, Init Angle/3
  Cos/1 -> Mux/2
  Memory/1 -> Sum/1
  Product/1 -> Conversion Rotation to Angle/1, Memory/1
  Memory1/1 -> Init Angle/1
  Init Angle/1 -> Sum1/3, Memory1/1

== system irp_model/Position 5/Filters 5 ==
  Sin && Cos : Inport
  Analog Butterworth LP Filter : Subsystem  mask(buttap){}
      mask help:
      | Analog Butterworth low pass filter.
      |
      | (Requires Signal Processing Toolbox)
      mask init:
      | [z,p,k]=buttap(@2); z=@1*z; p=@1*p; k=real(prod(-p)); [num,den]=zp2tf(z,p,k); w=logspace(log10(@1/10),log10(10*@1),20); h=freqs(num,den,w);
      mask Help: Butterworth low pass filter using MATLAB's butter command.
      mask Display: plot(20*log10(w),20*log10(abs(h)))
  Analog Butterworth LP Filter1 : Subsystem  mask(buttap){}
      mask help:
      | Analog Butterworth low pass filter.
      |
      | (Requires Signal Processing Toolbox)
      mask init:
      | [z,p,k]=buttap(@2); z=@1*z; p=@1*p; k=real(prod(-p)); [num,den]=zp2tf(z,p,k); w=logspace(log10(@1/10),log10(10*@1),20); h=freqs(num,den,w);
      mask Help: Butterworth low pass filter using MATLAB's butter command.
      mask Display: plot(20*log10(w),20*log10(abs(h)))
  Demux : Demux  Outputs=2
  Sin : Outport
  Cos : Outport  Port=2
  wires:
  Analog Butterworth LP Filter/1(Out1) -> Sin/1
  Analog Butterworth LP Filter1/1(Out1) -> Cos/1
  Sin && Cos/1 -> Demux/1
  Demux/1 -> Analog Butterworth LP Filter/1(In1)
  Demux/2 -> Analog Butterworth LP Filter1/1(In1)

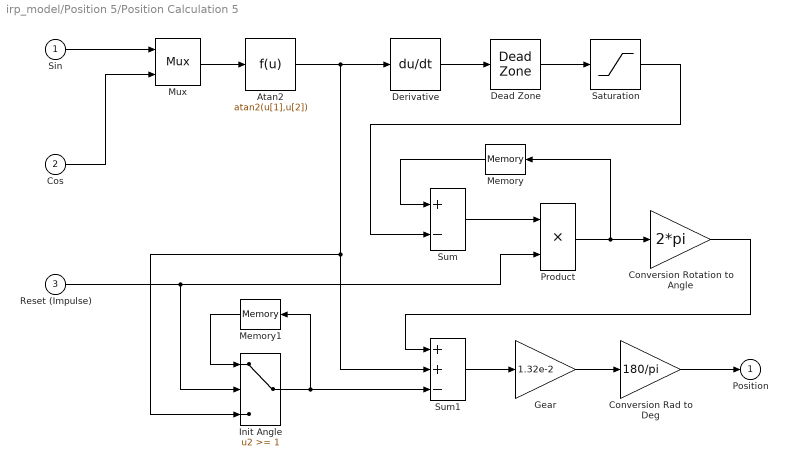
== system irp_model/Position 5/Position Calculation 5 ==
  Sin : Inport
  Cos : Inport  Port=2
  Reset (Impulse) : Inport  Port=3
  Atan2 : Fcn  Expr=atan2(u[1],u[2])
  Conversion Rad to Deg : Gain  Gain=180/pi  SaturateOnIntegerOverflow=on  OutDataTypeStr=Inherit: Same as input  ParamDataTypeStr=Inherit: Same as input
  Conversion Rotation to Angle : Gain  Gain=2*pi  SaturateOnIntegerOverflow=on  OutDataTypeStr=Inherit: Same as input  ParamDataTypeStr=Inherit: Same as input
  Dead Zone : DeadZone  LowerValue=-5000  UpperValue=5000  SaturateOnIntegerOverflow=on
  Derivative : Derivative
  Gear : Gain  Gain=1.32e-2  SaturateOnIntegerOverflow=on  OutDataTypeStr=Inherit: Same as input  ParamDataTypeStr=Inherit: Same as input
  Init Angle : Switch  Threshold=1  SaturateOnIntegerOverflow=on  InputSameDT=on
  Memory : Memory
  Memory1 : Memory
  Mux : Mux  Inputs=2
  Product : Product  SaturateOnIntegerOverflow=on  RndMeth=Zero  InputSameDT=on  OutDataTypeStr=Inherit: Same as first input
  Saturation : Saturate  UpperLimit=1  LowerLimit=-1
  Sum : Sum  Inputs=+-  SaturateOnIntegerOverflow=on  InputSameDT=on  OutDataTypeStr=Inherit: Same as first input
  Sum1 : Sum  Inputs=++-  SaturateOnIntegerOverflow=on  InputSameDT=on  OutDataTypeStr=Inherit: Same as first input
  Position : Outport
  wires:
  Gear/1 -> Conversion Rad to Deg/1
  Sum1/1 -> Gear/1
  Sum/1 -> Product/1
  Dead Zone/1 -> Saturation/1
  Derivative/1 -> Dead Zone/1
  Mux/1 -> Atan2/1
  Sin/1 -> Mux/1
  Conversion Rad to Deg/1 -> Position/1
  Saturation/1 -> Sum/2
  Conversion Rotation to Angle/1 -> Sum1/1
  Reset (Impulse)/1 -> Product/2, Init Angle/2
  Atan2/1 -> Derivative/1, Sum1/2, Init Angle/3
  Cos/1 -> Mux/2
  Memory/1 -> Sum/1
  Product/1 -> Conversion Rotation to Angle/1, Memory/1
  Memory1/1 -> Init Angle/1
  Init Angle/1 -> Sum1/3, Memory1/1

== system irp_model/Position 1/Filters 1/Analog Butterworth LP Filter ==
  In1 : Inport
  Analog Butterworth LP Filter : ZeroPole  Zeros=z  Poles=p  Gain=k
  Out1 : Outport
  wires:
  Analog Butterworth LP Filter/1 -> Out1/1
  In1/1 -> Analog Butterworth LP Filter/1

== system irp_model/Position 1/Filters 1/Analog Butterworth LP Filter1 ==
  In1 : Inport
  Analog Butterworth LP Filter1 : ZeroPole  Zeros=z  Poles=p  Gain=k
  Out1 : Outport
  wires:
  Analog Butterworth LP Filter1/1 -> Out1/1
  In1/1 -> Analog Butterworth LP Filter1/1

== system irp_model/Position 2/Filters 2/Analog Butterworth LP Filter ==
  In1 : Inport
  Analog Butterworth LP Filter : ZeroPole  Zeros=z  Poles=p  Gain=k
  Out1 : Outport
  wires:
  Analog Butterworth LP Filter/1 -> Out1/1
  In1/1 -> Analog Butterworth LP Filter/1

== system irp_model/Position 2/Filters 2/Analog Butterworth LP Filter1 ==
  In1 : Inport
  Analog Butterworth LP Filter1 : ZeroPole  Zeros=z  Poles=p  Gain=k
  Out1 : Outport
  wires:
  Analog Butterworth LP Filter1/1 -> Out1/1
  In1/1 -> Analog Butterworth LP Filter1/1

== system irp_model/Position 3/Filters 3/Analog Butterworth LP Filter ==
  In1 : Inport
  Analog Butterworth LP Filter : ZeroPole  Zeros=z  Poles=p  Gain=k
  Out1 : Outport
  wires:
  Analog Butterworth LP Filter/1 -> Out1/1
  In1/1 -> Analog Butterworth LP Filter/1

== system irp_model/Position 3/Filters 3/Analog Butterworth LP Filter1 ==
  In1 : Inport
  Analog Butterworth LP Filter1 : ZeroPole  Zeros=z  Poles=p  Gain=k
  Out1 : Outport
  wires:
  Analog Butterworth LP Filter1/1 -> Out1/1
  In1/1 -> Analog Butterworth LP Filter1/1

== system irp_model/Position 4/Filters 4/Analog Butterworth LP Filter ==
  In1 : Inport
  Analog Butterworth LP Filter : ZeroPole  Zeros=z  Poles=p  Gain=k
  Out1 : Outport
  wires:
  Analog Butterworth LP Filter/1 -> Out1/1
  In1/1 -> Analog Butterworth LP Filter/1

== system irp_model/Position 4/Filters 4/Analog Butterworth LP Filter1 ==
  In1 : Inport
  Analog Butterworth LP Filter1 : ZeroPole  Zeros=z  Poles=p  Gain=k
  Out1 : Outport
  wires:
  Analog Butterworth LP Filter1/1 -> Out1/1
  In1/1 -> Analog Butterworth LP Filter1/1

== system irp_model/Position 5/Filters 5/Analog Butterworth LP Filter ==
  In1 : Inport
  Analog Butterworth LP Filter : ZeroPole  Zeros=z  Poles=p  Gain=k
  Out1 : Outport
  wires:
  Analog Butterworth LP Filter/1 -> Out1/1
  In1/1 -> Analog Butterworth LP Filter/1

== system irp_model/Position 5/Filters 5/Analog Butterworth LP Filter1 ==
  In1 : Inport
  Analog Butterworth LP Filter1 : ZeroPole  Zeros=z  Poles=p  Gain=k
  Out1 : Outport
  wires:
  Analog Butterworth LP Filter1/1 -> Out1/1
  In1/1 -> Analog Butterworth LP Filter1/1
